simulink model "Simulation01"  (R2018a)
settings: Solver=VariableStepAuto  StartTime=0.0  StopTime=10.0  RelTol=1e-3
libraries: simulink x2
settings Model: Creator=dasun  LastModifiedBy=dasun

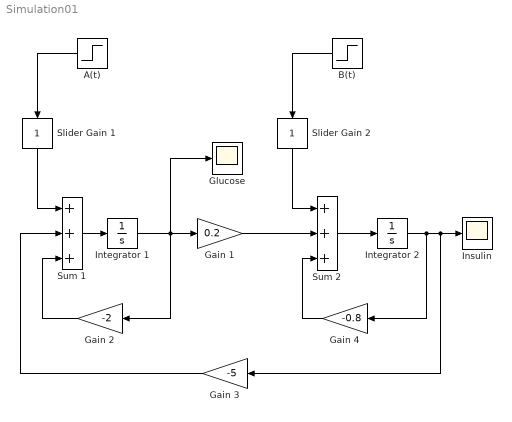
== system Simulation01 ==
  A(t) : Step  SampleTime=0
  B(t) : Step  After=0  SampleTime=0
  "Gain 1 " : Gain  Gain=0.2
  "Gain 2 " : Gain  Gain=-2
  "Gain 3 " : Gain  Gain=-5
  "Gain 4 " : Gain  Gain=-0.8
  Glucose : Scope
  Insulin : Scope
  "Integrator 1 " : Integrator
  "Integrator 2 " : Integrator
  Slider Gain 1 : simulink/Math Operations/Slider Gain  gain=1  low=0  high=2
  Slider Gain 2 : simulink/Math Operations/Slider Gain  gain=1  low=0  high=2
  Sum 1 : Sum  Inputs=+++
  "Sum 2 " : Sum  Inputs=+++
  wires:
  A(t)/1 -> Slider Gain 1/1
  B(t)/1 -> Slider Gain 2/1
  Slider Gain 1/1 -> Sum 1/1
  Sum 1/1 -> "Integrator 1 "/1
  "Integrator 1 "/1 -> "Gain 2 "/1, Glucose/1, "Gain 1 "/1
  "Gain 2 "/1 -> Sum 1/3
  "Gain 3 "/1 -> Sum 1/2
  "Gain 1 "/1 -> "Sum 2 "/2
  Slider Gain 2/1 -> "Sum 2 "/1
  "Gain 4 "/1 -> "Sum 2 "/3
  "Sum 2 "/1 -> "Integrator 2 "/1
  "Integrator 2 "/1 -> Insulin/1, "Gain 3 "/1, "Gain 4 "/1
